simulink model "sistem_termic_RF_model"  (R2025a)
settings: Solver=ode1be  StartTime=0.0  StopTime=Tfin  FixedStep=Ts  RelTol=1e-3
values from neighbouring files (symbols this model uses):
  f1 = 1/40/pi/5    (= 0.00159154943092)    [sistem_termic_RF_setup.m]
  f2 = 1/4/pi*5    (= 0.39788735773)    [sistem_termic_RF_setup.m]
  K = 1.2    [sistem_termic_RF_setup.m]
  T1 = 20    [sistem_termic_RF_setup.m]
  t1 = 10    [sistem_termic_RF_setup.m]
  T2 = 1.5    [sistem_termic_RF_setup.m]
  Tfin = 1500    [sistem_termic_RF_setup.m]
  Ts = 1e-1    (= 0.1)    [sistem_termic_RF_setup.m]
  u0 = 0    [sistem_termic_RF_setup.m]
  umax = 15    [sistem_termic_RF_setup.m]
  umin = -15    [sistem_termic_RF_setup.m]
  ust = 1    [sistem_termic_RF_setup.m]
  whtn_pow_in = 1e-6    (= 1e-06)    [sistem_termic_RF_setup.m]
  whtn_pow_out = 1e-6    (= 1e-06)    [sistem_termic_RF_setup.m]
  whtn_seed_in = 23341    [sistem_termic_RF_setup.m]
  whtn_seed_out = 23342    [sistem_termic_RF_setup.m]
  whtn_Ts_in = Ts    (= 0.1)    [sistem_termic_RF_setup.m]
  whtn_Ts_out = Ts    (= 0.1)    [sistem_termic_RF_setup.m]
  x0 = [7,0.1]    [sistem_termic_RF_setup.m]
  ymax = 15    [sistem_termic_RF_setup.m]
  ymin = -15    [sistem_termic_RF_setup.m]
libraries: simulink x5
settings Model: Creator=mircea  LastModifiedBy=mircea

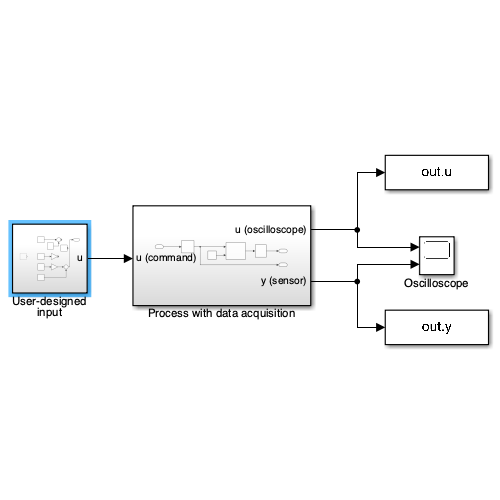
[thumbnail: Simulink's stored preview of the top-level diagram]
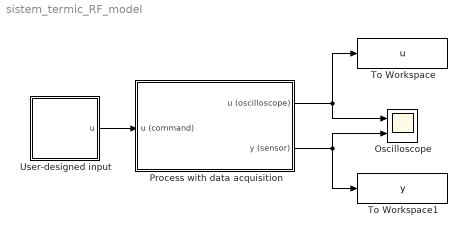
== system sistem_termic_RF_model ==
  Oscilloscope : Scope  NumInputPorts=2
      settings: ActiveDisplayYMinimum=-1.4999999999999996  ActiveDisplayYMaximum=13.5
  Process with data acquisition : Subsystem
  To Workspace : ToWorkspace  VariableName=u  SampleTime=Ts
  To Workspace1 : ToWorkspace  VariableName=y  SampleTime=Ts
  User-designed input : Subsystem
  wires:
  Process with data acquisition/1(u (oscilloscope)) -> Oscilloscope/1, To Workspace/1
  Process with data acquisition/2(y (sensor)) -> Oscilloscope/2, To Workspace1/1
  User-designed input/1(u) -> Process with data acquisition/1(u (command))

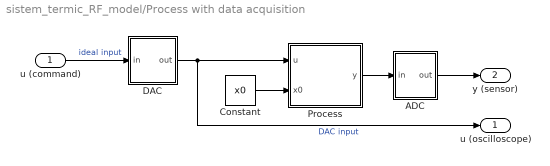
== system sistem_termic_RF_model/Process with data acquisition ==
  u (command) : Inport
  ADC : Subsystem
  Constant : Constant  Value=x0
  DAC : Subsystem
  Process : Subsystem
  u (oscilloscope) : Outport
  y (sensor) : Outport  Port=2
  wires:
  Constant/1 -> Process/2(x0)
  u (command)/1 -> DAC/1(in)  "ideal input"
  Process/1(y) -> ADC/1(in)
  ADC/1(out) -> y (sensor)/1
  DAC/1(out) -> Process/1(u), u (oscilloscope)/1  "DAC input"

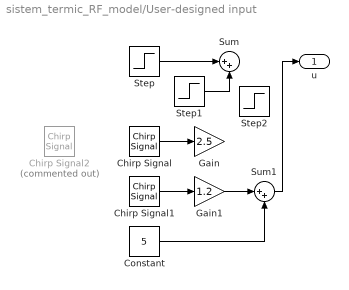
== system sistem_termic_RF_model/User-designed input ==
  Chirp Signal : simulink/Sources/Chirp Signal  f1=0.01  T=80  f2=15
  Chirp Signal1 : simulink/Sources/Chirp Signal  f1=f1/2  T=Tfin*1.1  f2=f2/5
  Chirp Signal2 : simulink/Sources/Chirp Signal  Commented=on  f1=1.9231e+03  T=1e-2  f2=1.0000e+04
  Constant : Constant  Value=5
  Gain : Gain  Gain=2.5
  Gain1 : Gain  Gain=1.2
  Step : Step  Time=5  Before=u0  After=ust  SampleTime=0
  Step1 : Step  Time=t1  Before=u0  After=ust  SampleTime=0
  Step2 : Step  Time=0  SampleTime=0
  Sum : Sum  Inputs=|++
  Sum1 : Sum  Inputs=|++
  u : Outport
  wires:
  Chirp Signal/1 -> Gain/1
  Step/1 -> Sum/1
  Step1/1 -> Sum/2
  Chirp Signal1/1 -> Gain1/1
  Gain1/1 -> Sum1/1
  Sum1/1 -> u/1
  Constant/1 -> Sum1/2

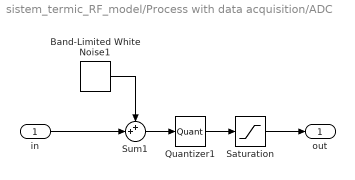
== system sistem_termic_RF_model/Process with data acquisition/ADC ==
  in : Inport
  Band-Limited White Noise1 : simulink/Sources/Band-Limited White Noise  Cov=[whtn_pow_out]  Ts=whtn_Ts_out  seed=[whtn_seed_out]
  Quantizer1 : Quantizer  QuantizationInterval=q_out
  Saturation : Saturate  UpperLimit=ymax  LowerLimit=ymin
  Sum1 : Sum  Inputs=++|
  out : Outport
  wires:
  Quantizer1/1 -> Saturation/1
  Sum1/1 -> Quantizer1/1
  in/1 -> Sum1/2
  Band-Limited White Noise1/1 -> Sum1/1
  Saturation/1 -> out/1

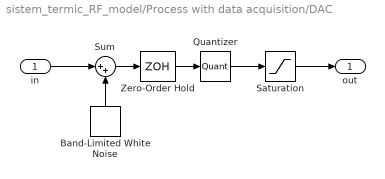
== system sistem_termic_RF_model/Process with data acquisition/DAC ==
  in : Inport
  Band-Limited White Noise : simulink/Sources/Band-Limited White Noise  Cov=[whtn_pow_in]  Ts=whtn_Ts_in  seed=[whtn_seed_in]
  Quantizer : Quantizer  QuantizationInterval=q_in
  Saturation : Saturate  UpperLimit=umax  LowerLimit=umin
  Sum : Sum  Inputs=|++
  Zero-Order Hold : ZeroOrderHold  SampleTime=-1
  out : Outport
  wires:
  Quantizer/1 -> Saturation/1
  Sum/1 -> Zero-Order Hold/1
  in/1 -> Sum/1
  Band-Limited White Noise/1 -> Sum/2
  Zero-Order Hold/1 -> Quantizer/1
  Saturation/1 -> out/1

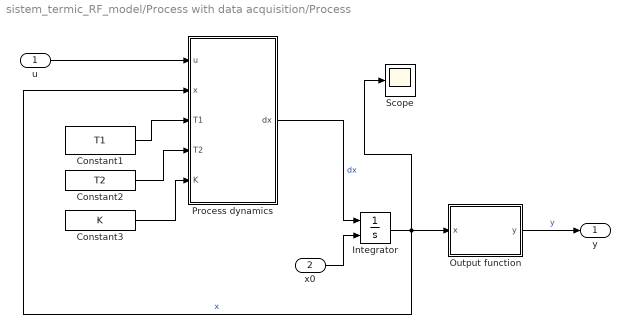
== system sistem_termic_RF_model/Process with data acquisition/Process ==
  u : Inport
  x0 : Inport  Port=2
  Constant1 : Constant  Value=T1
  Constant2 : Constant  Value=T2
  Constant3 : Constant  Value=K
  Integrator : Integrator  InitialConditionSource=external
  Output function : MATLAB Function  TreatAsAtomicUnit=on
  Process dynamics : MATLAB Function  TreatAsAtomicUnit=on
  Scope : Scope
      settings: ActiveDisplayYMinimum=-30864.820368316767  ActiveDisplayYMaximum=30756.992827113063
  y : Outport
  wires:
  u/1 -> Process dynamics/1(u)
  Process dynamics/1(dx) -> Integrator/1  "dx"
  Integrator/1 -> Scope/1, Output function/1(x), Process dynamics/2(x)  "x"
  Output function/1(y) -> y/1  "y"
  x0/1 -> Integrator/2
  Constant2/1 -> Process dynamics/4(T2)
  Constant1/1 -> Process dynamics/3(T1)
  Constant3/1 -> Process dynamics/5(K)

== matlab function sistem_termic_RF_model/Process with data acquisition/Process/Process dynamics ==
  data: u input; dx output; x input; T1 input; T2 input; K input
function dx = fcn(u,x,T1,T2,K)
dx = [0,1;
    -1/T1/T2,-(1/T1+1/T2)]*x + [0;K/T1/T2]*u;
end

== matlab function sistem_termic_RF_model/Process with data acquisition/Process/Output function ==
  data: y output; x input
function y = fcn(x)

y = x(1);

end
